simulink model "s_2dbb"  (R2020b)
settings: Solver=ode1  StartTime=0.0  StopTime=40  FixedStep=0.002  RelTol=1e-3  AbsTol=1e-6  EnableMultiTasking=on
values from neighbouring files (symbols this model uses):
  K_AMP = 1    [setup_2dbb.m]
  K_bb = 0    [setup_2dbb.m]
  kd = 0    [setup_2dbb.m]
  kp = 0    [setup_2dbb.m]
  VMAX_DAC = 10    [setup_2dbb.m]
  wf = 2 * pi * 2.5    (= 15.7079632679)    [setup_2dbb.m]
undefined symbols (not defined in the file or in its folder): K, tau, THETA_MAX, THETA_MIN, VMAX_AMP
libraries: simulink x1, simulink_extras x1
settings Model: ExtModeTrigDuration=25000  Creator=MLevis  LastModifiedBy=5470
settings SolverCC: AutoScaleAbsTol=off  PositivePriorityOrder=on
settings DataIOCC: SaveFormat=Array  SignalLoggingSaveFormat=ModelDataLogs  ReturnWorkspaceOutputs=off
settings OptimizationCC: BlockReduction=off  BooleanDataType=off  OptimizeBlockIOStorage=off  BufferReuse=off  GlobalBufferReuse=off  ExpressionFolding=off  ExpressionDepthLimit=2147483647  LocalBlockOutputs=off  InitFltsAndDblsToZero=on  LifeSpan=inf  OptimizeDataStoreBuffers=off  BusAssignmentInplaceUpdate=off
settings DebuggingCC: SaveWithParameterizedLinksMsg=none  UnderspecifiedInitializationDetection=Classic  MergeDetectMultiDrivingBlocksExec=none  SignalResolutionControl=TryResolveAllWithWarning  MultiTaskDSMMsg=warning  MultiTaskCondExecSysMsg=none  FcnCallInpInsideContextMsg=warning  StateNameClashWarn=warning  SFUnexpectedBacktrackingDiag=warning  SFNoUnconditionalDefaultTransitionDiag=warning  SFExecutionAtInitializationDiag=none  ArithmeticOperatorsInVariantConditions=warning
settings HardwareCC: ProdBitPerPointer=32  ProdBitPerSizeT=32  ProdBitPerPtrDiffT=32  ProdLargestAtomicFloat=None  ProdIntDivRoundTo=Undefined  ProdEndianess=Unspecified  ProdWordSize=32  ProdHWDeviceType=32-bit Generic  TargetHWDeviceType=32-bit Generic
settings ModelReferenceCC: PropagateSignalLabelsOutOfModel=off
settings SFSimCC: SimUseLocalCustomCode=off  CustomCodeUndefinedFunction=UseInterfaceOnly
settings RTWCC: Description=Quarc Win32 Target  SystemTargetFile=quarc_windows.tlc  TemplateMakefile=quarc_default_tmf  RTWUseLocalCustomCode=off
settings CodeAppCC: StateflowObjectComments=on
settings STFCustomTargetCC: TargetFcnLib=ansi_tfl_tmw.mat  TargetPreCompLibLocation=C:\PROGRA~3\QUARC\lib\2018b\windows\release  ConcurrentExecutionCompliant=off  SystemTargetFile=quarc_windows.tlc
settings GRTTargetCC: TargetFcnLib=ansi_tfl_tmw.mat  TargetPreCompLibLocation=C:\PROGRA~3\QUARC\lib\2018b\windows\release  TargetLangStandard=C89/C90 (ANSI)  ParMdlRefBuildCompliant=off  CompOptLevelCompliant=off  ConcurrentExecutionCompliant=off  CombineOutputUpdateFcns=off  MatFileLogging=off  GRTInterface=on  UseToolchainInfoCompliant=off  ExtMode=on  ExtModeMexFile=quarc_comm
settings ConfigComp: CovMetricSettings=dw  CovSaveCumulativeToWorkspaceVar=on  CovSaveSingleToWorkspaceVar=on  CovExternalEMLEnable=off

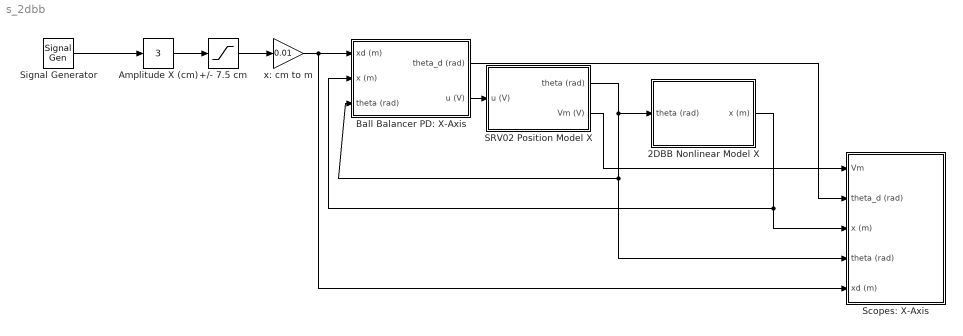
== system s_2dbb ==
  +/- 7.5 cm : Saturate  UpperLimit=7.5  LowerLimit=-7.5
  2DBB Nonlinear Model X : Subsystem
  Amplitude X (cm) : simulink/Math Operations/Slider Gain  gain=3  low=0  high=7.5
  Ball Balancer PD: X-Axis : Subsystem
  SRV02 Position Model X : Subsystem
  Scopes: X-Axis : Subsystem
  Signal Generator : SignalGenerator  WaveForm=square  Frequency=0.5  Units=rad/sec
  x: cm to m : Gain  Gain=0.01
  wires:
  Ball Balancer PD: X-Axis/2(u (V)) -> SRV02 Position Model X/1(u (V))
  SRV02 Position Model X/1(theta (rad)) -> 2DBB Nonlinear Model X/1(theta (rad)), Scopes: X-Axis/4(theta (rad)), Ball Balancer PD: X-Axis/3(theta (rad))
  Ball Balancer PD: X-Axis/1(theta_d (rad)) -> Scopes: X-Axis/2(theta_d (rad))
  2DBB Nonlinear Model X/1(x (m)) -> Ball Balancer PD: X-Axis/2(x (m)), Scopes: X-Axis/3(x (m))
  +/- 7.5 cm/1 -> x: cm to m/1
  Amplitude X (cm)/1 -> +/- 7.5 cm/1
  x: cm to m/1 -> Ball Balancer PD: X-Axis/1(xd (m)), Scopes: X-Axis/5(xd (m))
  SRV02 Position Model X/2(Vm (V)) -> Scopes: X-Axis/1(Vm)
  Signal Generator/1 -> Amplitude X (cm)/1

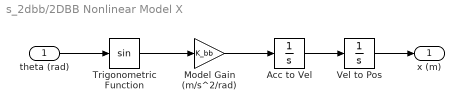
== system s_2dbb/2DBB Nonlinear Model X ==
  theta (rad) : Inport
  Acc to Vel : Integrator
  Model Gain (m/s^2/rad) : Gain  Gain=K_bb
  Trigonometric Function : Trigonometry
  Vel to Pos : Integrator
  x (m) : Outport  VectorParamsAs1DForOutWhenUnconnected=off
  wires:
  Trigonometric Function/1 -> Model Gain (m/s^2/rad)/1
  Acc to Vel/1 -> Vel to Pos/1
  Model Gain (m/s^2/rad)/1 -> Acc to Vel/1
  Vel to Pos/1 -> x (m)/1
  theta (rad)/1 -> Trigonometric Function/1

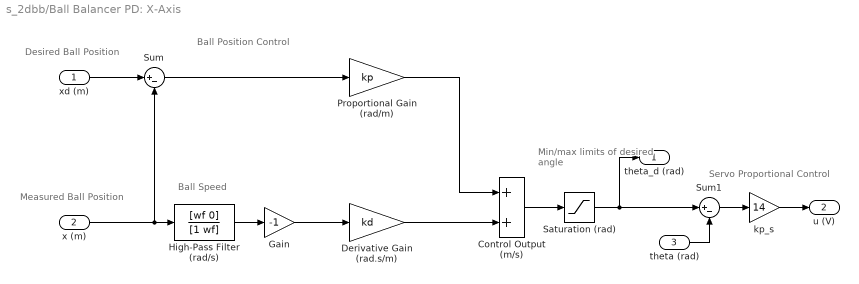
== system s_2dbb/Ball Balancer PD: X-Axis ==
  note: Ball Position Control
  note: Servo Proportional Control
  note: Min/max limits
      | of desired angle
  note: Desired Ball Position
  note: Measured Ball Position
  note: Ball Speed
  xd (m) : Inport
  x (m) : Inport  Port=2
  theta (rad) : Inport  Port=3
  Control Output (m/s) : Sum
  Derivative Gain (rad.s/m) : Gain  Gain=kd
  Gain : Gain  Gain=-1
  High-Pass Filter (rad/s) : TransferFcn  Numerator=[wf 0]  Denominator=[1 wf]
  Proportional Gain (rad/m) : Gain  Gain=kp
  Saturation (rad) : Saturate  UpperLimit=THETA_MAX  LowerLimit=THETA_MIN
  Sum : Sum  Inputs=|+-
  Sum1 : Sum  Inputs=|+-
  kp_s : Gain  Gain=14
  theta_d (rad) : Outport  VectorParamsAs1DForOutWhenUnconnected=off
  u (V) : Outport  Port=2  VectorParamsAs1DForOutWhenUnconnected=off
  wires:
  Derivative Gain (rad.s/m)/1 -> Control Output (m/s)/2
  kp_s/1 -> u (V)/1
  theta (rad)/1 -> Sum1/2
  Sum1/1 -> kp_s/1
  x (m)/1 -> Sum/2, High-Pass Filter (rad/s)/1
  Gain/1 -> Derivative Gain (rad.s/m)/1
  High-Pass Filter (rad/s)/1 -> Gain/1
  Sum/1 -> Proportional Gain (rad/m)/1
  xd (m)/1 -> Sum/1
  Control Output (m/s)/1 -> Saturation (rad)/1
  Saturation (rad)/1 -> theta_d (rad)/1, Sum1/1
  Proportional Gain (rad/m)/1 -> Control Output (m/s)/1

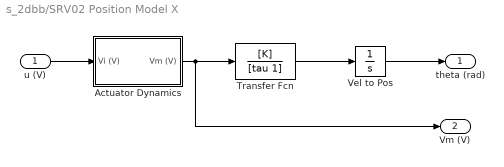
== system s_2dbb/SRV02 Position Model X ==
  u (V) : Inport
  Actuator Dynamics : Subsystem
  Transfer Fcn : TransferFcn  Numerator=[K]  Denominator=[tau 1]
  Vel to Pos : Integrator
  theta (rad) : Outport  VectorParamsAs1DForOutWhenUnconnected=off
  Vm (V) : Outport  Port=2  VectorParamsAs1DForOutWhenUnconnected=off
  wires:
  u (V)/1 -> Actuator Dynamics/1(Vi (V))
  Actuator Dynamics/1(Vm (V)) -> Vm (V)/1, Transfer Fcn/1
  Vel to Pos/1 -> theta (rad)/1
  Transfer Fcn/1 -> Vel to Pos/1

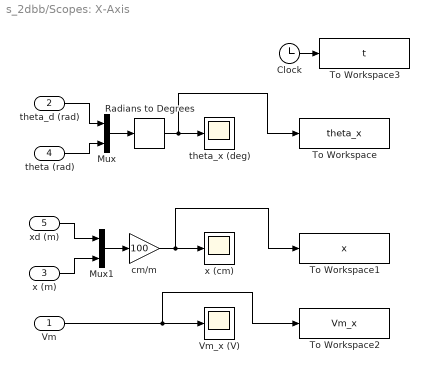
== system s_2dbb/Scopes: X-Axis ==
  Vm : Inport
  theta_d (rad) : Inport  Port=2
  x (m) : Inport  Port=3
  theta (rad) : Inport  Port=4
  xd (m) : Inport  Port=5
  Clock : Clock
  Mux : Mux  Inputs=2
  Mux1 : Mux  Inputs=2
  Radians to Degrees : simulink_extras/Transformations/Radians to Degrees
  To Workspace : ToWorkspace  VariableName=theta_x  SaveFormat=Timeseries  SampleTime=-1
  To Workspace1 : ToWorkspace  VariableName=x  SaveFormat=Timeseries  SampleTime=-1
  To Workspace2 : ToWorkspace  VariableName=Vm_x  SaveFormat=Timeseries  SampleTime=-1
  To Workspace3 : ToWorkspace  VariableName=t  SaveFormat=Timeseries  SampleTime=-1
  Vm_x (V) : Scope
  cm/m : Gain  Gain=100
  theta_x (deg) : Scope
  x (cm) : Scope
  wires:
  x (m)/1 -> Mux1/2
  xd (m)/1 -> Mux1/1
  Vm/1 -> To Workspace2/1, Vm_x (V)/1
  Radians to Degrees/1 -> To Workspace/1, theta_x (deg)/1
  Mux/1 -> Radians to Degrees/1
  Mux1/1 -> cm/m/1
  cm/m/1 -> To Workspace1/1, x (cm)/1
  theta (rad)/1 -> Mux/2
  theta_d (rad)/1 -> Mux/1
  Clock/1 -> To Workspace3/1

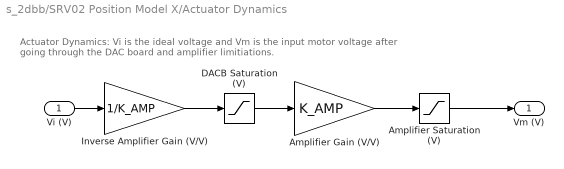
== system s_2dbb/SRV02 Position Model X/Actuator Dynamics ==
  note: Actuator Dynamics: Vi is the ideal voltage and Vm is the
      | input motor voltage after going through the DAC board and amplifier limitiations.
  Vi (V) : Inport
  Amplifier Gain (V/V) : Gain  Gain=K_AMP
  Amplifier Saturation (V) : Saturate  UpperLimit=VMAX_AMP  LowerLimit=-VMAX_AMP
  DACB Saturation (V) : Saturate  UpperLimit=VMAX_DAC  LowerLimit=-VMAX_DAC
  Inverse Amplifier Gain (V/V) : Gain  Gain=1/K_AMP
  Vm (V) : Outport  VectorParamsAs1DForOutWhenUnconnected=off
  wires:
  Amplifier Saturation (V)/1 -> Vm (V)/1
  Vi (V)/1 -> Inverse Amplifier Gain (V/V)/1
  Amplifier Gain (V/V)/1 -> Amplifier Saturation (V)/1
  DACB Saturation (V)/1 -> Amplifier Gain (V/V)/1
  Inverse Amplifier Gain (V/V)/1 -> DACB Saturation (V)/1
